simulink model "boostObserver"  (R2020a)
settings: Solver=ode45  StartTime=0.0  StopTime=1  FixedStep=0.0005  AbsTol=1e-06  EnableMultiTasking=on
InitFcn:
  | kp=0.01;
  | ki=0.01;
  | 
  | k=2;
  | em=100000000;
  | GE=1/em;
  | GU=k*ki/GE;
  | GCE=k*kp/GU;
model workspace (MAT data in the model file):
  time = 0.8
values from neighbouring files (symbols this model uses):
  A1 = obj.boostConverter.A1    [BoostController.m]    (also in BoostConverter.m = [-obj.R/obj.L 0;0 -1/(obj.Ro*obj.C)]; BuckBoostConverter.m = [-obj.R/obj.L 0;0 -1/(obj.Ro*obj.C)]; obsmc.m = Asigma{1,1}; workspace_atual.mat = [-16.4  0; 0  -3.50877192982])
  A2 = obj.boostConverter.A2    [BoostController.m]    (also in BoostConverter.m = [-obj.R/obj.L -1/obj.L;1/obj.C -1/(obj.Ro*obj.C)]; BuckBoostConverter.m = [-obj.R/obj.L 1/obj.L;-1/obj.C -1/(obj.Ro*obj.C)]; obsmc.m = Asigma{1,2}; workspace_atual.mat = [-16.4  -200; 350.877192982  -3.50877192982])
  B1 = obj.boostConverter.B1    [BoostController.m]    (also in BoostConverter.m = [1/obj.L;0]; BuckBoostConverter.m = [1/obj.L;0]; obsmc.m = Bsigma{1,1}; workspace_atual.mat = [200 0])
  c = 0.00285    [workspace_atual.mat]    (also in workspace_certo.mat)
  Cmatrix = [1  0; 0  1]    [workspace_atual.mat]    (also in workspace_certo.mat)
  Kg = [-8 -0.8 -2.3]    [workspace_atual.mat]    (also in workspace_certo.mat)
  Lnew1 = [0.000426144297292  -1.37628182296; -0.636691353583  10000.3869597]    [workspace_atual.mat]    (also in workspace_certo.mat = [0.00144628510103  0.00148492117427; 0.000288596381821  0.00)
  Lnew2 = [0.000454345330516  -0.588943865675; 0.999552025739  4999.94512306]    [workspace_atual.mat]    (also in workspace_certo.mat = [0.00251672143174  0.00251025627081; 6.60131109739e-05  6.53)
  LoadAddFactor = 0.30    (= 0.3)    [BoostFaultSimulation.m]    (also in workspace_atual.mat; workspace_certo.mat)
  LoadRemoveFactor = 0.30    (= 0.3)    [BoostFaultSimulation.m]    (also in workspace_atual.mat; workspace_certo.mat)
  R = 0.1    [boostResults2Latex.m]    (also in workspace_atual.mat = 0.082; workspace_certo.mat = 0.082)
  Ro = 100    [BoostFaultSimulation.m]    (also in boostResults2Latex.m = 10; workspace_atual.mat; workspace_certo.mat)
  Smep = 80    [workspace_atual.mat]    (also in workspace_certo.mat)
  SmFrequency = 7000    [workspace_atual.mat]    (also in workspace_certo.mat)
  SmiLGain = 8    [workspace_atual.mat]    (also in workspace_certo.mat)
  SmIntegralGain = 2.3    [workspace_atual.mat]    (also in workspace_certo.mat)
  SmVcGain = 0.8    [workspace_atual.mat]    (also in workspace_certo.mat)
  SourceAddFactor = 0.10    (= 0.1)    [BoostFaultSimulation.m]    (also in workspace_atual.mat; workspace_certo.mat)
  SourceAddSwitch = 0    [BoostFaultSimulation.m]    (also in workspace_atual.mat; workspace_certo.mat)
  SourceRemoveFactor = 0.10    (= 0.1)    [BoostFaultSimulation.m]    (also in workspace_atual.mat; workspace_certo.mat)
  Ts = 0.0001    [workspace_atual.mat]    (also in workspace_certo.mat)
  ueq = 0.5    [workspace_atual.mat]    (also in workspace_certo.mat)
  x_e = [ie;ve]    [BoostConverter.m]    (also in BuckBoostConverter.m)
  xe = obj.boostConverter.equilibriumstate(ve)    [BoostController.m]    (also in workspace_atual.mat = [7.62509288104 380]; workspace_certo.mat = [7.62509288104 380])
libraries: PhdLibrary x14, powerlib_meascontrol x2, eePwmGenerator x1
settings Model: SimulationMode=accelerator  Creator=d13go  LastModifiedBy=vitor
settings SolverCC: MaxConsecutiveZCs=10000  ZeroCrossAlgorithm=Adaptive  DecoupledContinuousIntegration=on  MinimalZcImpactIntegration=on
settings DataIOCC: SaveFinalState=on  SaveState=on  LoggingToFile=on
settings OptimizationCC: DefaultParameterBehavior=Inlined  UseDivisionForNetSlopeComputation=on  GainParamInheritBuiltInType=on  UseFloatMulNetSlope=on  InlineInvariantSignals=on  EfficientFloat2IntCast=on  LifeSpan=1
settings DebuggingCC: ReadBeforeWriteMsg=DisableAll  WriteAfterWriteMsg=DisableAll  WriteAfterReadMsg=DisableAll  AlgebraicLoopMsg=error  MaxConsecutiveZCsMsg=warning  MaskedZcDiagnostic=none  IgnoredZcDiagnostic=none  MultiTaskDSMMsg=none  SFUnexpectedBacktrackingDiag=warning  SFNoUnconditionalDefaultTransitionDiag=warning  ArithmeticOperatorsInVariantConditions=warning
settings HardwareCC: ProdLongLongMode=on
settings ModelReferenceCC: UpdateModelReferenceTargets=IfOutOfDate
settings SFSimCC: SFSimEcho=off  SimUseLocalCustomCode=off  MATLABDynamicMemAlloc=off  CustomCodeUndefinedFunction=UseInterfaceOnly
settings RTWCC: GenerateReport=on  RTWUseLocalCustomCode=off  LaunchReport=on
settings CodeAppCC: ForceParamTrailComments=on
settings GRTTargetCC: TargetLangStandard=C89/C90 (ANSI)  CombineSignalStateStructs=on  MatFileLogging=off  SupportVariableSizeSignals=on
settings ConfigComp: CovMetricSettings=dw  CovHtmlReporting=on  CovSaveCumulativeToWorkspaceVar=on  CovSaveSingleToWorkspaceVar=on  CovExternalEMLEnable=off
settings SimscapeCC: SimscapeNormalizeSystem=off

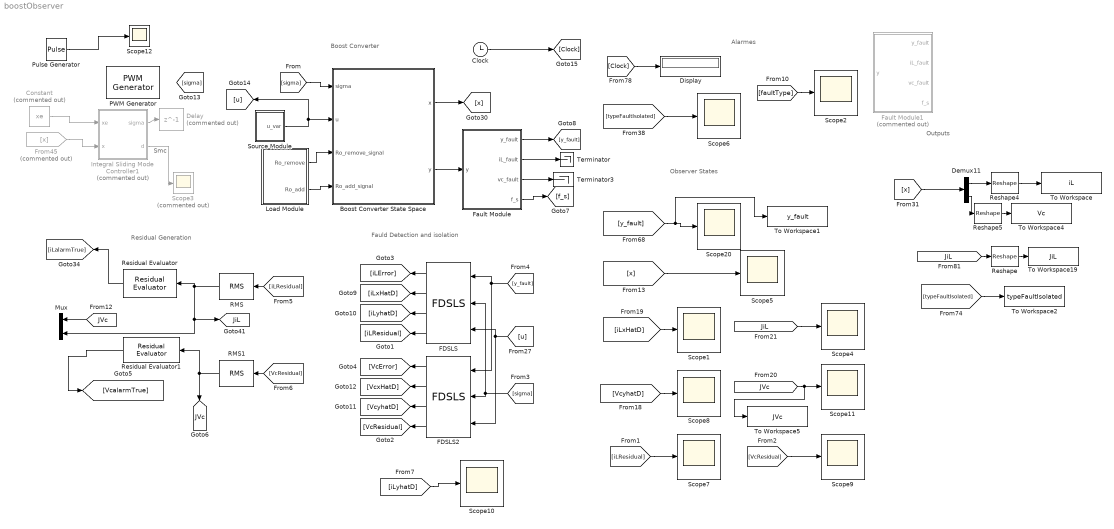
== system boostObserver ==
  note: Alarmes
  note: Smc
  note: Fauld Detection and isolation
  note: Outputs
  note: Observer States
  note: Residual Generation
  note: Boost Converter
  Boost Converter State Space : Subsystem  AncestorBlock="PhdLibrary/Boost Converter  State Space"  mask(Boots State-Space model){A1=A1, A2=A2, B1=B1, R=R, Ro=Ro, Cmatrix=Cmatrix, c=c, LoadAddFactor=LoadAddFactor, LoadRemoveFactor=LoadRemoveFactor}
      mask prompts: A1 "A1 matrix:"; A2 "A2 matrix:"; B1 "B matrix:"; R "Resistance:"; Ro "Output Resistance:"; Cmatrix "Output Matrix:"; c "Capacitance:"; LoadAddFactor "Load add factor:"; LoadRemoveFactor "Load remove factor"
      mask help: Boots State-Space model
      mask Display: disp('Boost')
  Clock : Clock
  Constant : Constant  Commented=on  Value=xe  VectorParams1D=off
  Delay : Delay  Commented=on  DelayLength=1
  Demux11 : Demux  Outputs=2
  Display : Display
  FDSLS : PhdLibrary/FDSLS  A1=A1  A2=A2  B1=B1  B2=B2  L=Lnew1  yhat0=[0;0]  x0=[0;0]  Qr=[1 0]
      link override Constant3: Value=Lnew1
      settings: SourceProductName=Phd Diego
  FDSLS2 : PhdLibrary/FDSLS  A1=A1  A2=A2  B1=B1  B2=B2  L=Lnew2  yhat0=[0;0]  x0=[0;0]  Qr=[0 1]
      link override Constant3: Value=Lnew2
      settings: SourceProductName=Phd Diego
  Fault Module : Subsystem
  Fault Module1 : Subsystem  Commented=on
  From45 : From  Commented=on  GotoTag=x
  Integral Sliding Mode Controller1 : Subsystem  Commented=on  mask(Sliding mode controller){KiVc=SmIntegralGain, KVc=SmVcGain, ueq=ueq, Smep=Smep, KiL=SmiLGain, Freq=SmFrequency, x0=[0;0], Ts=0}
      mask prompts: KiVc "Integral voltage gain"; KVc "Voltage gain"; ueq "Equilibrium signal"; Smep "Surface limit layer"; KiL "Current gain"; Freq "Frequency"; x0 "Initial state:"; Ts "Sample Time"
      mask help: Sliding mode controller with integral for boost converter
  Load Module : Subsystem
  Mux : Mux  Inputs=2
  PWM Generator : eePwmGenerator/PWM Generator  CarrCount=Up  Tper=1  Ts=5e-6
  Pulse Generator : DiscretePulseGenerator  Period=1  SampleTime=0.000005
  RMS : powerlib_meascontrol/Measurements/RMS  TrueRMS=on  Freq=RMSfrequency  RMSInit=0  Ts=Ts
  RMS1 : powerlib_meascontrol/Measurements/RMS  TrueRMS=on  Freq=RMSfrequency  RMSInit=0  Ts=Ts
  Reshape : Reshape
  Reshape4 : Reshape
  Reshape5 : Reshape
  Residual Evaluator : PhdLibrary/Residual Evaluator  Jth=iLJth
      settings: SourceProductName=Phd Diego
  Residual Evaluator1 : PhdLibrary/Residual Evaluator  Jth=VcJth
      settings: SourceProductName=Phd Diego
  Scope{1..2,4..12,20} (12 alike) : Scope
  Scope3 : Scope  Commented=on
  Source Module : Subsystem
  Terminator : Terminator
  Terminator3 : Terminator
  To Workspace : ToWorkspace  VariableName=iL  SaveFormat=Timeseries  SampleTime=-1
  To Workspace1 : ToWorkspace  VariableName=y_fault  SaveFormat=Timeseries  SampleTime=-1
  To Workspace19 : ToWorkspace  VariableName=JiL  SaveFormat=Timeseries  SampleTime=-1
  To Workspace2 : ToWorkspace  VariableName=typeFaultIsolated  SaveFormat=Timeseries  SampleTime=-1
  To Workspace4 : ToWorkspace  VariableName=Vc  SaveFormat=Timeseries  SampleTime=-1
  To Workspace5 : ToWorkspace  VariableName=JVc  SaveFormat=Timeseries  SampleTime=-1
  tag scope: JVc=global, JiL=global
  wires:
  [y_fault] -> FDSLS2/1, FDSLS/1
  [iLResidual] -> RMS/1
  [faultType] -> Scope2/1
  Clock/1 -> [Clock]
  Boost Converter State Space/1(x) -> [x]
  Fault Module/2(iL_fault) -> Terminator/1
  [JVc] -> To Workspace5/1, Scope11/1
  Load Module/1(Ro_remove) -> Boost Converter State Space/3(Ro_remove_signal)
  Residual Evaluator/1 -> [iLalarmTrue]
  Residual Evaluator1/1 -> [VcalarmTrue]
  [y_fault] -> To Workspace1/1, Scope20/1
  [JiL] -> Scope4/1
  [x] -> Demux11/1
  FDSLS2/2 -> [VcxHatD]
  Load Module/2(Ro_add) -> Boost Converter State Space/4(Ro_add_signal)
  Source Module/1(u_var) -> [u], Boost Converter State Space/2(u)
  Fault Module/4(f_s) -> [f_s]
  Boost Converter State Space/2(y) -> Fault Module/1(y)
  [VcResidual] -> RMS1/1
  [sigma] -> FDSLS2/2, FDSLS/2
  Demux11/1 -> Reshape4/1
  RMS1/1 -> Residual Evaluator1/1, [JVc]
  RMS/1 -> [JiL], Mux/2, Residual Evaluator/1
  [sigma] -> Boost Converter State Space/1(sigma)
  [x] -> Scope5/1
  FDSLS/4 -> [iLResidual]
  FDSLS2/3 -> [VcyhatD]
  Reshape4/1 -> To Workspace/1
  FDSLS2/1 -> [VcError]
  [VcyhatD] -> Scope8/1
  FDSLS/3 -> [iLyhatD]
  Fault Module/3(vc_fault) -> Terminator3/1
  Demux11/2 -> Reshape5/1
  FDSLS/1 -> [iLError]
  [typeFaultIsolated] -> To Workspace2/1
  [u] -> FDSLS2/3, FDSLS/3
  FDSLS2/4 -> [VcResidual]
  Fault Module/1(y_fault) -> [y_fault]
  [typeFaultIsolated] -> Scope6/1
  [JiL] -> Reshape/1
  Reshape/1 -> To Workspace19/1
  Reshape5/1 -> To Workspace4/1
  [Clock] -> Display/1
  [iLxHatD] -> Scope1/1
  FDSLS/2 -> [iLxHatD]
  [JVc] -> Mux/1
  Integral Sliding Mode Controller1/2(d) -> Scope3/1
  Constant/1 -> Integral Sliding Mode Controller1/1(xe)
  From45/1 -> Integral Sliding Mode Controller1/2(x)
  Integral Sliding Mode Controller1/1(sigma) -> Delay/1
  [iLResidual] -> Scope7/1
  [VcResidual] -> Scope9/1
  [iLyhatD] -> Scope10/1
  ? -> PWM Generator/1
  Pulse Generator/1 -> Scope12/1

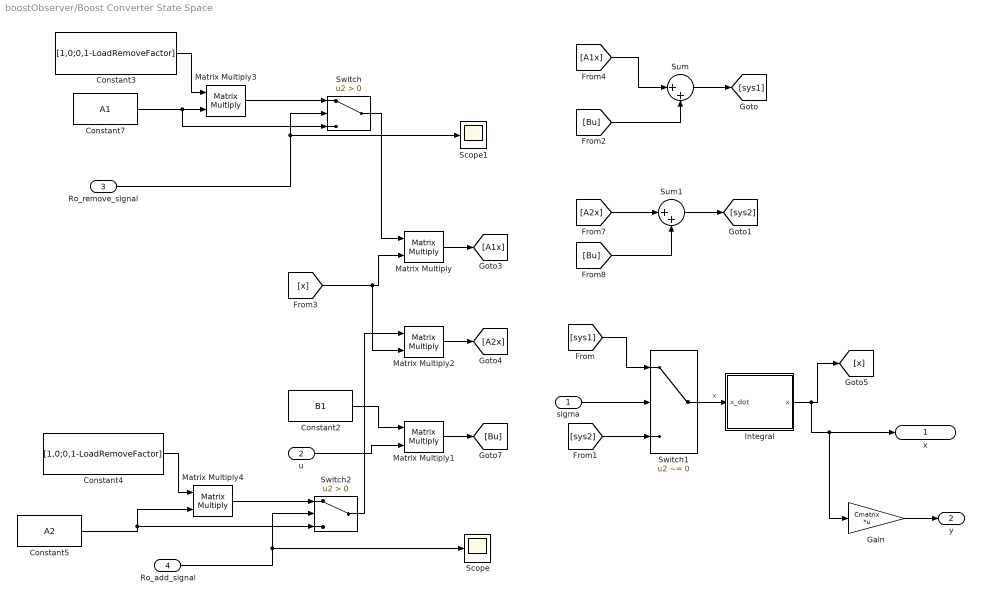
== system boostObserver/Boost Converter State Space ==
  sigma : Inport
  u : Inport  Port=2
  Ro_remove_signal : Inport  Port=3
  Ro_add_signal : Inport  Port=4
  Constant2 : Constant  Value=B1  VectorParams1D=off
  Constant3 : Constant  Value=[1,0;0,1-LoadRemoveFactor]  VectorParams1D=off
  Constant4 : Constant  Value=[1,0;0,1-LoadRemoveFactor]  VectorParams1D=off
  Constant5 : Constant  Value=A2  VectorParams1D=off
  Constant7 : Constant  Value=A1  VectorParams1D=off
  Gain : Gain  Gain=Cmatrix  Multiplication=Matrix(K*u)
  Integral : Subsystem
  Matrix Multiply{,1..4} (5 alike) : Product  Multiplication=Matrix(*)
  Scope : Scope
  Scope1 : Scope
  Sum : Sum  Inputs=|++
  Sum1 : Sum  Inputs=|++
  Switch : Switch  Criteria=u2 > Threshold
  Switch1 : Switch  Criteria=u2 ~= 0
  Switch2 : Switch  Criteria=u2 > Threshold
  x : Outport
  y : Outport  Port=2
  wires:
  Switch2/1 -> Matrix Multiply2/1
  Ro_add_signal/1 -> Scope/1, Switch2/2
  Constant5/1 -> Matrix Multiply4/2, Switch2/3
  Matrix Multiply4/1 -> Switch2/1
  Constant4/1 -> Matrix Multiply4/1
  Switch/1 -> Matrix Multiply/1
  Ro_remove_signal/1 -> Scope1/1, Switch/2
  Matrix Multiply3/1 -> Switch/1
  Constant7/1 -> Switch/3, Matrix Multiply3/2
  Constant3/1 -> Matrix Multiply3/1
  Gain/1 -> y/1
  Integral/1(x) -> [x], x/1, Gain/1
  u/1 -> Matrix Multiply1/2
  Matrix Multiply1/1 -> [Bu]
  Constant2/1 -> Matrix Multiply1/1
  sigma/1 -> Switch1/2
  [A2x] -> Sum1/1
  Switch1/1 -> Integral/1(x_dot)  "x"
  Sum1/1 -> [sys2]
  Sum/1 -> [sys1]
  Matrix Multiply/1 -> [A1x]
  Matrix Multiply2/1 -> [A2x]
  [Bu] -> Sum/2
  [Bu] -> Sum1/2
  [x] -> Matrix Multiply/2, Matrix Multiply2/2
  [A1x] -> Sum/1
  [sys1] -> Switch1/1
  [sys2] -> Switch1/3

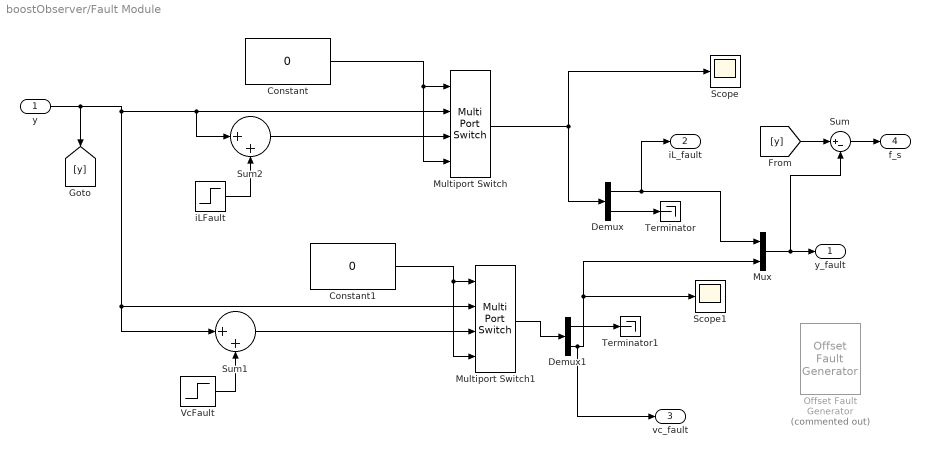
== system boostObserver/Fault Module ==
  y : Inport
  Constant : Constant  Value=0
  Constant1 : Constant  Value=0
  Demux : Demux  Outputs=2
  Demux1 : Demux  Outputs=2
  Multiport Switch : MultiPortSwitch  DataPortOrder=Zero-based contiguous  Inputs=2  DataPortForDefault=Additional data port  zeroidx=on
  Multiport Switch1 : MultiPortSwitch  DataPortOrder=Zero-based contiguous  Inputs=2  DataPortForDefault=Additional data port  zeroidx=on
  Mux : Mux  Inputs=2
  Offset Fault Generator : PhdLibrary/Offset Fault Generator  Commented=on  s1gain=20  s2gain=20
      settings: SourceProductName=Phd Diego
  Scope : Scope
  Scope1 : Scope
  Sum : Sum  Inputs=|+-
  Sum1 : Sum  Inputs=|++
  Sum2 : Sum  Inputs=|++
  Terminator : Terminator
  Terminator1 : Terminator
  VcFault : Step  Time=0.5  After=50  SampleTime=0
  iLFault : Step  Time=0.5  After=2  SampleTime=0
  y_fault : Outport
  iL_fault : Outport  Port=2
  vc_fault : Outport  Port=3
  f_s : Outport  Port=4
  wires:
  y/1 -> Multiport Switch1/2, Sum1/1, Sum2/1, Multiport Switch/2, [y]
  Constant/1 -> Multiport Switch/1, Multiport Switch/4
  Constant1/1 -> Multiport Switch1/1, Multiport Switch1/4
  Multiport Switch/1 -> Scope/1, Demux/1
  Multiport Switch1/1 -> Demux1/1
  Demux/2 -> Terminator/1
  Demux/1 -> iL_fault/1, Mux/1
  Mux/1 -> Sum/2, y_fault/1
  Demux1/1 -> Terminator1/1
  Demux1/2 -> vc_fault/1, Mux/2, Scope1/1
  [y] -> Sum/1
  Sum/1 -> f_s/1
  VcFault/1 -> Sum1/2
  Sum1/1 -> Multiport Switch1/3
  Sum2/1 -> Multiport Switch/3
  iLFault/1 -> Sum2/2

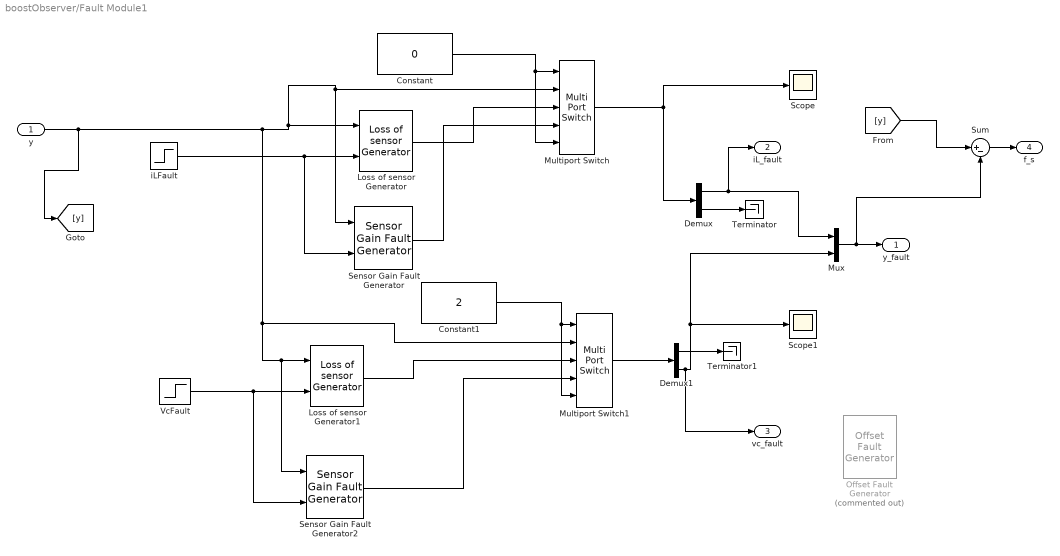
== system boostObserver/Fault Module1 ==
  y : Inport
  Constant : Constant  Value=0
  Constant1 : Constant  Value=2
  Demux : Demux  Outputs=2
  Demux1 : Demux  Outputs=2
  Loss of sensor Generator : PhdLibrary/Loss of sensor Generator
      settings: SourceProductName=Phd Diego
  Loss of sensor Generator1 : PhdLibrary/Loss of sensor Generator
      settings: SourceProductName=Phd Diego
  Multiport Switch : MultiPortSwitch  DataPortOrder=Zero-based contiguous  DataPortForDefault=Additional data port  zeroidx=on
  Multiport Switch1 : MultiPortSwitch  DataPortOrder=Zero-based contiguous  DataPortForDefault=Additional data port  zeroidx=on
  Mux : Mux  Inputs=2
  Offset Fault Generator : PhdLibrary/Offset Fault Generator  Commented=on  s1gain=20  s2gain=20
      settings: SourceProductName=Phd Diego
  Scope : Scope
  Scope1 : Scope
  Sensor Gain Fault Generator : PhdLibrary/Sensor Gain Fault Generator  s1gain=iLGainFaultFactor  s2gain=VcGainFaultFactor
      settings: SourceProductName=Phd Diego
  Sensor Gain Fault Generator2 : PhdLibrary/Sensor Gain Fault Generator  s1gain=iLGainFaultFactor  s2gain=VcGainFaultFactor
      settings: SourceProductName=Phd Diego
  Sum : Sum  Inputs=|+-
  Terminator : Terminator
  Terminator1 : Terminator
  VcFault : Step  Time=0.5  After=2  SampleTime=0
  iLFault : Step  Time=0.5  SampleTime=0
  y_fault : Outport
  iL_fault : Outport  Port=2
  vc_fault : Outport  Port=3
  f_s : Outport  Port=4
  wires:
  iLFault/1 -> Sensor Gain Fault Generator/2, Loss of sensor Generator/2
  y/1 -> [y], Multiport Switch1/2, Sensor Gain Fault Generator2/1, Loss of sensor Generator1/1, Sensor Gain Fault Generator/1, Multiport Switch/2, Loss of sensor Generator/1
  VcFault/1 -> Sensor Gain Fault Generator2/2, Loss of sensor Generator1/2
  Constant/1 -> Multiport Switch/5, Multiport Switch/1
  Constant1/1 -> Multiport Switch1/5, Multiport Switch1/1
  Multiport Switch/1 -> Scope/1, Demux/1
  Multiport Switch1/1 -> Demux1/1
  Demux/2 -> Terminator/1
  Demux/1 -> iL_fault/1, Mux/1
  Mux/1 -> Sum/2, y_fault/1
  Demux1/1 -> Terminator1/1
  Demux1/2 -> vc_fault/1, Mux/2, Scope1/1
  Loss of sensor Generator/1 -> Multiport Switch/3
  Sensor Gain Fault Generator/1 -> Multiport Switch/4
  Sensor Gain Fault Generator2/1 -> Multiport Switch1/4
  Loss of sensor Generator1/1 -> Multiport Switch1/3
  [y] -> Sum/1
  Sum/1 -> f_s/1

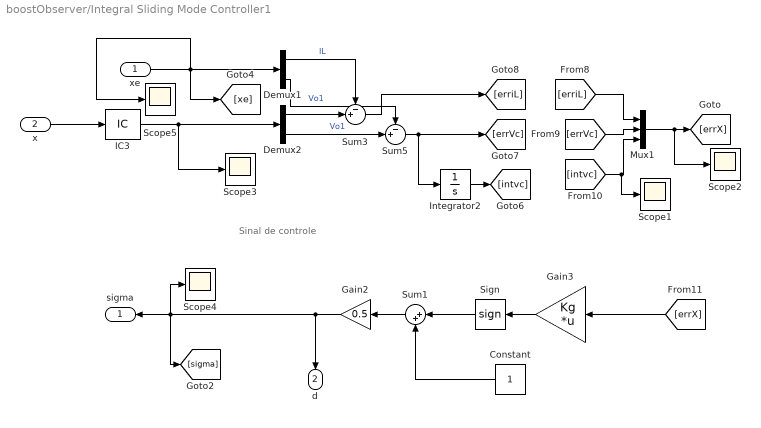
== system boostObserver/Integral Sliding Mode Controller1 ==
  note: Sinal de controle
  xe : Inport
  x : Inport  Port=2
  Constant : Constant
  Demux1 : Demux  Outputs=2
  Demux2 : Demux  Outputs=2
  Gain2 : Gain  Gain=0.5
  Gain3 : Gain  Gain=Kg  Multiplication=Matrix(K*u)
  IC3 : InitialCondition  Value=x0
  Integrator2 : Integrator
  Mux1 : Mux  Inputs=3
  Scope{1..5} (5 alike) : Scope
  Sign : Signum
  Sum1 : Sum  Inputs=|++
  Sum3 : Sum  Inputs=-+|
  Sum5 : Sum  Inputs=-+|
  sigma : Outport
  d : Outport  Port=2
  wires:
  IC3/1 -> Scope3/1, Demux2/1
  xe/1 -> [xe], Scope5/1, Demux1/1
  x/1 -> IC3/1
  Sum1/1 -> Gain2/1
  Constant/1 -> Sum1/2
  Demux1/2 -> Sum5/1  "Vo1"
  Demux2/2 -> Sum5/2  "Vo1"
  Sum5/1 -> Integrator2/1, [errVc]
  Demux1/1 -> Sum3/1  "IL"
  Demux2/1 -> Sum3/2
  Sum3/1 -> [erriL]
  Integrator2/1 -> [intvc]
  [erriL] -> Mux1/1
  [errVc] -> Mux1/2
  [intvc] -> Scope1/1, Mux1/3
  Mux1/1 -> Scope2/1, [errX]
  Gain2/1 -> [sigma], Scope4/1, sigma/1, d/1
  Gain3/1 -> Sign/1
  Sign/1 -> Sum1/1
  [errX] -> Gain3/1

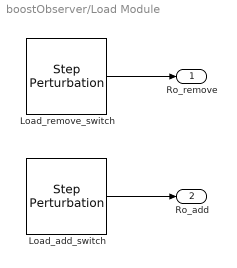
== system boostObserver/Load Module ==
  Load_add_switch : PhdLibrary/Step Perturbation  SignalSwitch=LoadAddSignalSwitch  InitialMagnitude=0  InitialTime=LoadAddTime  Magnitude=1  Duration=LoadAddDuration  enabled=LoadAddSwitch
      settings: SourceProductName=Phd Diego
  Load_remove_switch : PhdLibrary/Step Perturbation  SignalSwitch=LoadRemoveSignalSwitch  InitialMagnitude=0  InitialTime=LoadRemoveTime  Magnitude=1  Duration=LoadRemoveDuration  enabled=LoadRemoveSwitch
      settings: SourceProductName=Phd Diego
  Ro_remove : Outport
  Ro_add : Outport  Port=2
  wires:
  Load_remove_switch/1 -> Ro_remove/1
  Load_add_switch/1 -> Ro_add/1

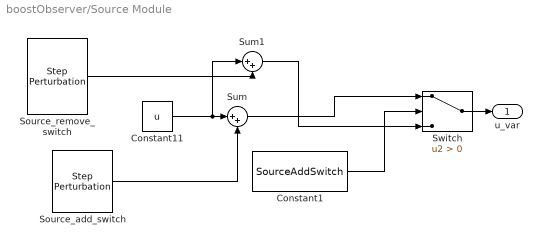
== system boostObserver/Source Module ==
  Constant1 : Constant  Value=SourceAddSwitch  VectorParams1D=off
  Constant11 : Constant  Value=u
  Source_add_switch : PhdLibrary/Step Perturbation  SignalSwitch=SourceAddSignalSwitch  InitialMagnitude=0  InitialTime=SourceAddTime  Magnitude=SourceAddFactor*u  Duration=SourceAddDuration  enabled=SourceAddSwitch
      settings: SourceProductName=Phd Diego
  Source_remove_switch : PhdLibrary/Step Perturbation  SignalSwitch=SourceRemoveSignalSwitch  InitialMagnitude=0  InitialTime=SourceRemoveTime  Magnitude=-SourceRemoveFactor*u  Duration=SourceRemoveDuration  enabled=SourceRemoveSwitch
      settings: SourceProductName=Phd Diego
  Sum : Sum  Inputs=|++
  Sum1 : Sum  Inputs=|++
  Switch : Switch  Criteria=u2 > Threshold
  u_var : Outport
  wires:
  Sum1/1 -> Switch/3
  Sum/1 -> Switch/1
  Constant11/1 -> Sum1/1, Sum/1
  Switch/1 -> u_var/1
  Source_add_switch/1 -> Sum/2
  Source_remove_switch/1 -> Sum1/2
  Constant1/1 -> Switch/2

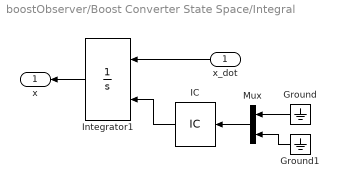
== system boostObserver/Boost Converter State Space/Integral ==
  x_dot : Inport
  Ground : Ground
  Ground1 : Ground
  IC : InitialCondition  Value=[0;0]
  Integrator1 : Integrator  InitialConditionSource=external  InitialCondition=[-x_e; 0; 0]
  Mux : Mux  Inputs=2
  x : Outport
  wires:
  Mux/1 -> IC/1
  Ground/1 -> Mux/1
  Ground1/1 -> Mux/2
  IC/1 -> Integrator1/2
  Integrator1/1 -> x/1
  x_dot/1 -> Integrator1/1
